simulink model "LAB0_2"  (R2024b)
settings: Solver=VariableStepAuto  StartTime=0.0  StopTime=45  FixedStep=0.001  RelTol=1e-3
undefined symbols (not defined in the file or in its folder): degs2rpm, den_Hi, den_Hw, gbox, Kd_opt, Ki_opt, Kp_opt, mot, num_Hi, num_Hw, rpm2degs, sens, Tl
libraries: simulink x1
settings Model: Creator=Gioele  LastModifiedBy=Gioele
settings DataIOCC: ReturnWorkspaceOutputs=off
settings ConfigComp: CovBoundaryAbsTol=1.0e-5

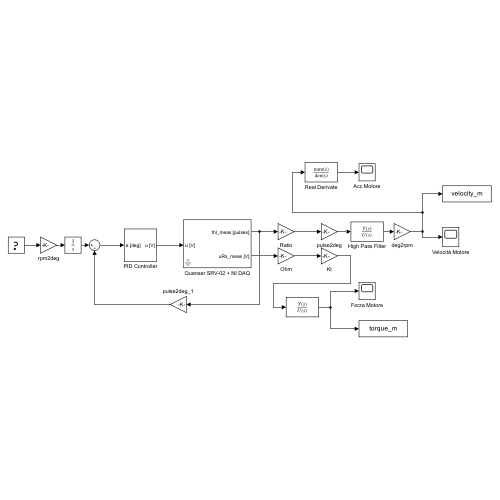
[thumbnail: Simulink's stored preview of the top-level diagram]
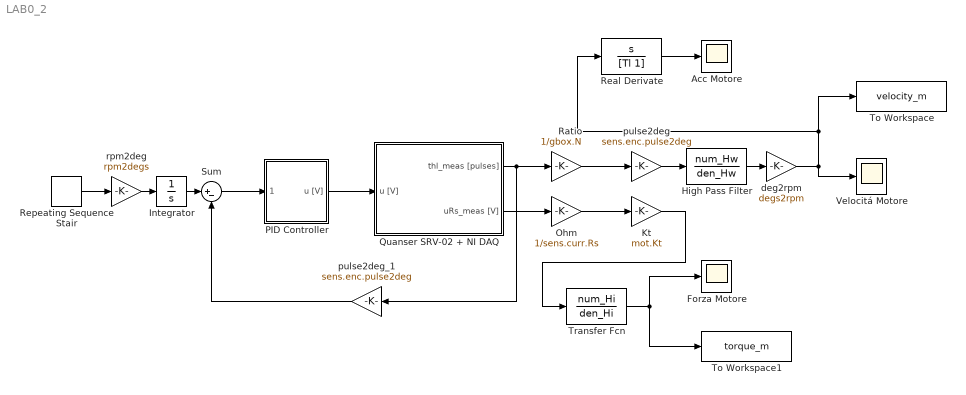
== system LAB0_2 ==
  Acc Motore : Scope
  Forza Motore : Scope
  High Pass Filter : TransferFcn  Numerator=num_Hw  Denominator=den_Hw
  Integrator : Integrator
  Kt : Gain  Gain=mot.Kt
  Ohm : Gain  Gain=1/sens.curr.Rs
  PID Controller : Subsystem
  Quanser SRV-02 + NI DAQ : Subsystem  mask(Quanser SRV-02 (with inertial load) + NI DAQ){Ts=0.001, fricType=Coulomb + viscous}
      mask prompts: Ts "NI DAQ Sample Time:"; fricType "Friction model"
      mask help: Quanser SRV-02 (with inertial load) + NI DAQ model.
      mask init:
      | %%  Sensors data
      | 
      | %   shunt resistor
      | sens.curr.Rs = 0.5;                         %   resistance [Ohm]   
      | sens.curr.uRs_std = 0.01;                   %   voltage noise standard dev [V]                           
      | sens.curr.uRs_var = sens.curr.uRs_std^2;	%   voltage noise variance [V^2]
      | 
      | %   Hewlett-Packard HEDS-5540#A06 optical encoder
      | sens.enc.ppr = 500*4;                       %   pulses per rotation
      | sens.enc.pulse2deg = 360/sens.enc.ppr;      %   [pulses] -> [deg]
      | sens.enc.pulse2rad = 2*pi/sens.enc.ppr;     %   [pulses] -> [rad]
      | sens.enc.deg2pulse = sens.enc.ppr/360;      %   [deg] -> [pulses]
      | sens.enc.rad2pulse = sens.enc.ppr/2/pi;     %   [rad] -> [pulses]
      | 
      | 
      | %%  Data acquisition board (daq) data
      | 
      | %   NI PCI-6221 DAC data
      | daq.dac.bits = 16;                                  %   resolution (bits)
      | daq.dac.fs   = 10;                                  %   full scale 
      | daq.dac.q    = 2*daq.dac.fs/(2^daq.dac.bits-1);     %	quantization
      | 
      | %   NI PCI-6221 ADC data
      | daq.adc.bits = 16;                                  %   resolution (bits)
      | daq.adc.fs   = 10;                                  %   full scale (as set in SLDRT Analog Input block)
      | daq.adc.q    = 2*daq.adc.fs/(2^daq.adc.bits-1);     %   quantization
      mask Help:
      | Riccardo Antonello (antonello@dei.unipd.it)
      | 
      | April 24, 2020
      | 
      | Dept. of Information Engineering, University of Padova
      mask TypeOptions fricType: Coulomb + viscous | Karnopp
  Ratio : Gain  Gain=1/gbox.N
  Real Derivate : TransferFcn  Numerator=[1 0]  Denominator=[Tl 1]
  Repeating Sequence Stair : simulink/Sources/Repeating Sequence Stair  OutValues=stair_rpm  tsamp=5  OutMin=[]  OutMax=[]  OutDataTypeStr=double  OutputDataTypeScalingMode=double  OutDataType=fixdt(0,8)  ConRadixGroup=Best Precision: Vector-wise  OutScaling=2^-12
  Sum : Sum  Inputs=|+-
  To Workspace : ToWorkspace  VariableName=velocity_m  SaveFormat=Timeseries  SampleTime=-1
  To Workspace1 : ToWorkspace  VariableName=torque_m  SaveFormat=Timeseries  SampleTime=-1
  Transfer Fcn : TransferFcn  Numerator=num_Hi  Denominator=den_Hi
  Velocitá Motore : Scope
  deg2rpm : Gain  Gain=degs2rpm
  pulse2deg : Gain  Gain=sens.enc.pulse2deg
  pulse2deg_1 : Gain  Gain=sens.enc.pulse2deg
  rpm2deg : Gain  Gain=rpm2degs
  wires:
  PID Controller/1(u [V]) -> Quanser SRV-02 + NI DAQ/1(u [V])
  Sum/1 -> PID Controller/1(e [deg])
  pulse2deg_1/1 -> Sum/2
  Quanser SRV-02 + NI DAQ/1(thl_meas [pulses]) -> pulse2deg_1/1, Ratio/1
  Quanser SRV-02 + NI DAQ/2(uRs_meas [V]) -> Ohm/1
  Ohm/1 -> Kt/1
  Kt/1 -> Transfer Fcn/1
  Repeating Sequence Stair/1 -> rpm2deg/1
  Integrator/1 -> Sum/1
  Transfer Fcn/1 -> Forza Motore/1, To Workspace1/1
  Ratio/1 -> pulse2deg/1
  rpm2deg/1 -> Integrator/1
  pulse2deg/1 -> High Pass Filter/1
  High Pass Filter/1 -> deg2rpm/1
  deg2rpm/1 -> To Workspace/1, Real Derivate/1, Velocitá Motore/1
  Real Derivate/1 -> Acc Motore/1

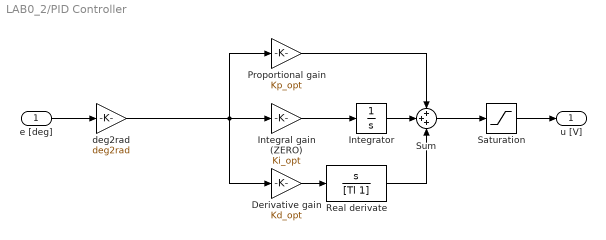
== system LAB0_2/PID Controller ==
  e [deg] : Inport
  Derivative gain : Gain  Gain=Kd_opt
  Integral gain (ZERO) : Gain  Gain=Ki_opt
  Integrator : Integrator
  Proportional gain : Gain  Gain=Kp_opt
  Real derivate : TransferFcn  Numerator=[1 0]  Denominator=[Tl 1]
  Saturation : Saturate  UpperLimit=10  LowerLimit=-10
  Sum : Sum  Inputs=+++
  deg2rad : Gain  Gain=deg2rad
  u [V] : Outport
  wires:
  e [deg]/1 -> deg2rad/1
  Saturation/1 -> u [V]/1
  Sum/1 -> Saturation/1
  Integrator/1 -> Sum/2
  Derivative gain/1 -> Real derivate/1
  Proportional gain/1 -> Sum/1
  deg2rad/1 -> Proportional gain/1, Derivative gain/1, Integral gain (ZERO)/1
  Integral gain (ZERO)/1 -> Integrator/1
  Real derivate/1 -> Sum/3

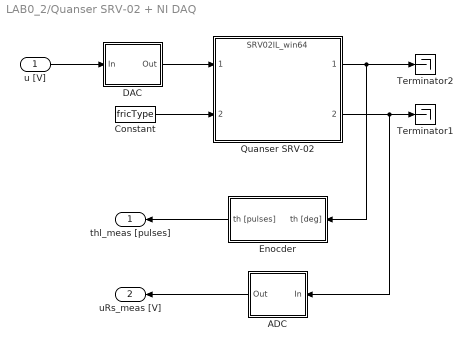
== system LAB0_2/Quanser SRV-02 + NI DAQ ==
  u [V] : Inport
  ADC : Subsystem
  Constant : Constant  Value=fricType
  DAC : Subsystem
  Enocder : Subsystem
  Quanser SRV-02 : ModelReference  ModelNameDialog=SRV02IL_win64.slxp  ModelReferenceVersion=1.44  CopyOfModelProtected=on
  Terminator1 : Terminator
  Terminator2 : Terminator
  thl_meas [pulses] : Outport
  uRs_meas [V] : Outport  Port=2
  wires:
  Enocder/1(th [pulses]) -> thl_meas [pulses]/1
  ADC/1(Out) -> uRs_meas [V]/1
  DAC/1(Out) -> Quanser SRV-02/1
  Quanser SRV-02/2 -> ADC/1(In), Terminator1/1
  u [V]/1 -> DAC/1(In)
  Quanser SRV-02/1 -> Enocder/1(th [deg]), Terminator2/1
  Constant/1 -> Quanser SRV-02/2

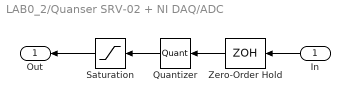
== system LAB0_2/Quanser SRV-02 + NI DAQ/ADC ==
  In : Inport
  Quantizer : Quantizer  QuantizationInterval=daq.adc.q
  Saturation : Saturate  UpperLimit=daq.adc.fs  LowerLimit=-daq.adc.fs
  Zero-Order Hold : ZeroOrderHold  SampleTime=Ts
  Out : Outport
  wires:
  Saturation/1 -> Out/1
  In/1 -> Zero-Order Hold/1
  Quantizer/1 -> Saturation/1
  Zero-Order Hold/1 -> Quantizer/1

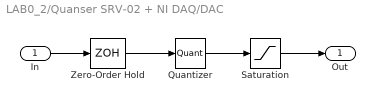
== system LAB0_2/Quanser SRV-02 + NI DAQ/DAC ==
  In : Inport
  Quantizer : Quantizer  QuantizationInterval=daq.dac.q
  Saturation : Saturate  UpperLimit=daq.dac.fs  LowerLimit=-daq.dac.fs
  Zero-Order Hold : ZeroOrderHold  SampleTime=Ts
  Out : Outport
  wires:
  Quantizer/1 -> Saturation/1
  In/1 -> Zero-Order Hold/1
  Zero-Order Hold/1 -> Quantizer/1
  Saturation/1 -> Out/1

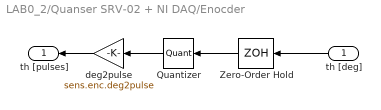
== system LAB0_2/Quanser SRV-02 + NI DAQ/Enocder ==
  th [deg] : Inport
  Quantizer : Quantizer  QuantizationInterval=sens.enc.pulse2deg
  Zero-Order Hold : ZeroOrderHold  SampleTime=Ts
  deg2pulse : Gain  Gain=sens.enc.deg2pulse
  th [pulses] : Outport
  wires:
  Quantizer/1 -> deg2pulse/1
  th [deg]/1 -> Zero-Order Hold/1
  Zero-Order Hold/1 -> Quantizer/1
  deg2pulse/1 -> th [pulses]/1
